simulink model "controls_project"  (R2021b)
settings: Solver=VariableStepAuto  StartTime=0.0  StopTime=0.1  RelTol=1e-3
model workspace (MAT data in the model file):
  Kb = Simulink.Parameter
  Kb.Value = 0.333333333333
  Kb.Description = 'wheel angle (beta) gain'
  Kb.DataType = 'auto'
  Kb.Complexity = 'real'
  Kb.Dimensions = [1 1]
  Ke = Simulink.Parameter
  Ke.Value = 0.001
  Ke.Description = 'electrical torque'
  Ke.DataType = 'auto'
  Ke.Complexity = 'real'
  Ke.Dimensions = [1 1]
  Kg = Simulink.Parameter
  Kg.Value = 0.016
  Kg.DataType = 'auto'
  Kg.Complexity = 'real'
  Kg.Dimensions = [1 1]
  Kt = Simulink.Parameter
  Kt.Value = 0.0174800008535
  Kt.Description = 'motor torque constant'
  Kt.DataType = 'auto'
  Kt.Complexity = 'real'
  Kt.Dimensions = [1 1]
  L = Simulink.Parameter
  L.Value = 7.67110577726e-06
  L.Description = 'phase inductance'
  L.DataType = 'auto'
  L.Complexity = 'real'
  L.Dimensions = [1 1]
  R = Simulink.Parameter
  R.Value = 0.0229220949113
  R.Description = 'phase resistance'
  R.DataType = 'auto'
  R.Complexity = 'real'
  R.Dimensions = [1 1]
  Te = Simulink.Parameter
  Te.Value = 0.0001156
  Te.Description = 'electrical constant'
  Te.DataType = 'auto'
  Te.Complexity = 'real'
  Te.Dimensions = [1 1]
  Tm = Simulink.Parameter
  Tm.Value = 0.0175
  Tm.Description = 'mechanical constant
    | '
  Tm.DataType = 'auto'
  Tm.Complexity = 'real'
  Tm.Dimensions = [1 1]
libraries: simulink_extras x1
settings Model: Creator=rcmas  LastModifiedBy=rcmas

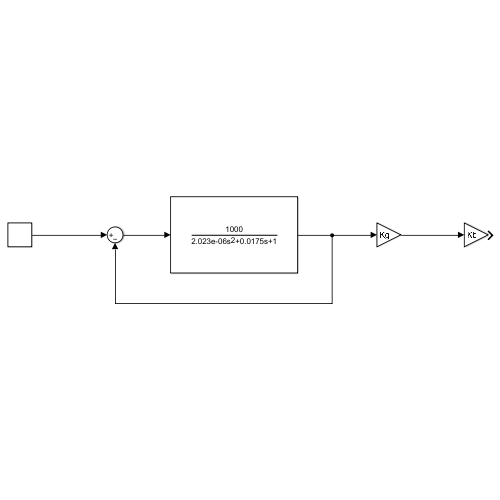
[thumbnail: Simulink's stored preview of the top-level diagram]
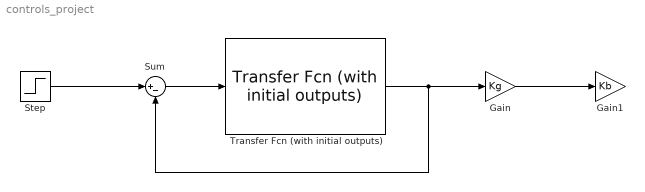
== system controls_project ==
  Gain : Gain  Gain=Kg
  Gain1 : Gain  Gain=Kb
  Step : Step  Time=0  After=50  SampleTime=0
  Sum : Sum  Inputs=|+-
  Transfer Fcn (with initial outputs) : simulink_extras/Additional Linear/Transfer Fcn (with initial outputs)  N=[1/Ke]  D=[Tm*Te Tm 1]  Y0=0  U0=0
  wires:
  Transfer Fcn (with initial outputs)/1 -> Sum/2, Gain/1
  Gain/1 -> Gain1/1
  Step/1 -> Sum/1
  Sum/1 -> Transfer Fcn (with initial outputs)/1
